simulink model "MenakaModel"  (R2022a)
settings: Solver=ode23tb  StartTime=0.0  StopTime=4  MaxStep=10/(60*24)  RelTol=1e-3
model workspace (MAT data in the model file):
  clima__A_c = 3295.16408265
  clima__A_f = 3100.53942116
  clima__G0 = [0.05; 0.00070738]
  clima__H = 7.9995824611
  clima__T0 = [287.15; 287.15; 287.15; 287.15]
  clima__T_ss = 280.150340169
  clima__alpha_c = 0.0100640347387
  clima__alpha_f = 0.0111385012129
  clima__alpha_i = 0.1
  clima__c_s = [1081 1081]
  clima__cd_c = 8736
  clima__d_c = 1.5
  clima__hour0 = 1
  clima__int_air_speed = 0.5
  clima__l_s = [0.1 0.1]
  clima__lam_s = [2.5 0.85]
  clima__minWindows = 0.299965865643
  clima__rhod_s = [2600 2500]
  clima__tau_c = 1
  crop__A_v = 2080
  crop__C = [0.01 0.001 0.01 0.01]
  crop__C_buf_max = 0.02
  crop__C_wv = 0.2
  crop__Chi_nutrients = [0.015625; 0.0104166666667; 0.00520833333333; 0.00208333333333; 0.00208333333333; 0.00104166666667; 0; 0]
  crop__N = [0; 0; 0; 0; 0; 0; 0; 0]
  crop__R = [0 0 0]
  crop__T_max_v = 40
  crop__T_max_v24 = 27
  crop__T_min_v = 6
  crop__T_min_v24 = 14
  crop__T_sum_end = 1035
  crop__T_v_start_fruit = 1100
  crop__Tsum = 0
  crop__Tv = 288
  crop__b_N_uptake = 0.5
  crop__c_fruit_g = 0.27
  crop__c_fruit_m = 2.3e-07
  crop__c_leaf_g = 0.28
  crop__c_leaf_m = 3.47e-07
  crop__c_stem_g = 0.3
  crop__c_stem_m = 1.47e-07
  crop__fraction_DM = 0.08
  crop__int_air_speed = 0.5
  crop__min_water_capacity = 0.1
  crop__plants_density = 2.1562
  crop__rg_fruit = 2e-07
  crop__rg_leaf = 9.5e-08
  crop__rg_stem = 7.4e-08
  crop__s_buforg_buf = -5000
  crop__s_max_T = 0.5793
  crop__s_max_T24 = 1.3904
  crop__s_min_T = -0.869
  crop__s_min_T24 = -1.1587
  heater__A_e = 0.0001
  heater__A_i = 0.008
  heater__T = 288
  heater__c = 5e-10
  heater__power = 60000000
  screen__Power = 100
  screen__Radthreshold = 900
  screen__beta = 2.23564167038e-14
  screen__gamma_max = 2.26308905438e-14
  screen__velocity = 0.333333333333
  subtrate__C_ws = 0.1
  subtrate__N = [0; 0; 0; 0; 0; 0; 0; 0]
  subtrate__Nmin_subs = 1e-09
  subtrate__Vmax_subs = 10
  subtrate__Vmin_subs = 0.01
  subtrate__sigma_max = 1
  subtrate__sigma_min = 1
  tomato__Cfruit0 = 0.001
  windows__AR = 19.9974923936
  windows__Power = 100
  windows__RadThreshold = 10
  windows__max_night = 10
  windows__tau = 600
undefined symbols (not defined in the file or in its folder): CO2_ppm_ext, Gain_control_Tv_mean, Gain_control_Tv_mean_superior, gain_max_night, GAIN_WIN, Hmax, Hstart, max_night, maxvelocity, RadTh_windows, Radthhold, shift_temp_heat, tau_win, tend_crop1, tend_crop2, tinit_crop1, tinit_crop2, Tmax, Tmax_mean, Tstart, Tven_max, Tven_start, WinAR
libraries: HORTISIM x26, simulink x6
(part 3 of 5)

== system MenakaModel/Control System/Control System Proportional (Ti) + Tmu Windows Relay/Heating Controler/Subsystem2 ==
  " Min" : Inport
  Max : Inport  Port=2
  T : Inport  Port=3
  Divide : Product  Inputs=*/
  Gain : Gain  Gain=0.5
  Gain1 : Gain  Gain=0.5
  Minus : Sum  Inputs=+-
  Minus1 : Sum  Inputs=+-
  Saturation : Saturate  UpperLimit=1  LowerLimit=0
  Sum : Sum  Inputs=|++
  y : Outport
  wires:
  Saturation/1 -> y/1
  Max/1 -> Gain1/1
  T/1 -> Minus/1
  Minus1/1 -> Divide/2
  Minus/1 -> Divide/1
  Divide/1 -> Saturation/1
  " Min"/1 -> Gain/1, Minus1/1
  Gain/1 -> Sum/1
  Gain1/1 -> Sum/2
  Sum/1 -> [Tmu]
  [Tmu] -> Minus1/2, Minus/2

== system MenakaModel/Control System/Control System Proportional (Ti) + Tmu Windows Relay/Screen Controler/Subsystem ==
  In1 : Inport
  Radthhold : Inport  Port=2
  If : If  IfExpression=u1 < 10
  If Action Subsystem : Subsystem  TreatAsAtomicUnit=on
  If Action Subsystem1 : Subsystem  TreatAsAtomicUnit=on
  Merge : Merge
  Smooth Rad : Subsystem
  Out1 : Outport
  wires:
  If/2 -> If Action Subsystem1/Action
  Smooth Rad/1(Out1) -> If/1
  If Action Subsystem1/1(Out1) -> Merge/2
  Merge/1 -> Out1/1
  In1/1 -> If Action Subsystem1/1(EC), Smooth Rad/1(In1)
  If/1 -> If Action Subsystem/Action
  If Action Subsystem/1(Out1) -> Merge/1
  Radthhold/1 -> If Action Subsystem1/2(Radthhold)

== system MenakaModel/Control System/Control System Proportional (Ti) + Tmu Windows Relay/Subsystem/Scalar2Bus  ==
  QV : Inport
  QT : Inport  Port=2
  A : Inport  Port=3
  CC : Inport  Port=4
  Bus Creator : BusCreator  Inputs=4
  CoCl : Outport
  wires:
  A/1 -> Bus Creator/3  "A"
  CC/1 -> Bus Creator/4  "CC"
  QV/1 -> Bus Creator/1  "QV"
  Bus Creator/1 -> CoCl/1
  QT/1 -> Bus Creator/2  "QT"

== system MenakaModel/Control System/Control System Proportional (Ti) + Tmu Windows Relay/Windows Controler/Subsystem ==
  Tstart : Inport
  Ti : Inport  Port=2
  Tmax : Inport  Port=3
  HRInt : Inport  Port=4
  HRStart : Inport  Port=5
  HRMax : Inport  Port=6
  Rad : Inport  Port=7
  Constant : Constant  Value=RadThreshold
  Hum : Saturate  UpperLimit=max_night  LowerLimit=0
  "Selection " : MATLAB Function  TreatAsAtomicUnit=on
  Subsystem : Subsystem
  Temp : Saturate  UpperLimit=100  LowerLimit=0
  Ventilation by Hight Humidity : MATLAB Function  TreatAsAtomicUnit=on
  y : Outport
  wires:
  Ti/1 -> Subsystem/2(Ti)
  Rad/1 -> "Selection "/1(Rad)
  Tstart/1 -> Subsystem/1(Tstart)
  Hum/1 -> "Selection "/3(Humidity)
  HRMax/1 -> Ventilation by Hight Humidity/3(HRMax)
  Tmax/1 -> Subsystem/3(Tmax)
  "Selection "/1(y) -> y/1
  Ventilation by Hight Humidity/1(y) -> Hum/1
  HRStart/1 -> Ventilation by Hight Humidity/2(HRStart)
  Subsystem/1(y) -> Temp/1
  HRInt/1 -> Ventilation by Hight Humidity/1(HRInt)
  Temp/1 -> "Selection "/2(Temperature)
  Constant/1 -> "Selection "/4(Rad_threshold)

== system MenakaModel/Control System/ON//OFF - constant setpoints/Subsystem/Scalar2Bus  ==
  QV : Inport
  QT : Inport  Port=2
  A : Inport  Port=3
  CC : Inport  Port=4
  Bus Creator : BusCreator  Inputs=4
  CoCl : Outport
  wires:
  A/1 -> Bus Creator/3  "A"
  CC/1 -> Bus Creator/4  "CC"
  QV/1 -> Bus Creator/1  "QV"
  Bus Creator/1 -> CoCl/1
  QT/1 -> Bus Creator/2  "QT"

== system MenakaModel/Control System/ON//OFF - constant setpoints/Subsystem1/From Temperature To Heater ST ==
  Tmax : Inport
  Tmin : Inport  Port=2
  Tmean : Inport  Port=3
  Constant1 : Constant  Value=shift_temp_heat
  Constant2 : Constant  Value=shift_temp_heat
  Integrator : Integrator  InitialConditionSource=external
  Minus2 : Sum  Inputs=+-
  Sum : Sum  Inputs=|++
  Sum1 : Sum  Inputs=|++
  Tmax_h : Outport
  Tstart_h : Outport  Port=2
  Tplus : Outport  Port=3
  Tminus : Outport  Port=4
  T_mu_mu : Outport  Port=5
  tag scope: Tmax_heater=global, Tmin_heater=global
  wires:
  Tmax/1 -> Sum/1
  Sum/1 -> [Tmax_heater], Tmax_h/1
  Tmin/1 -> Sum1/1
  Sum1/1 -> Tstart_h/1, [Tmin_heater]
  Constant1/1 -> Sum/2
  Constant2/1 -> Sum1/2
  Integrator/1 -> Minus2/2, T_mu_mu/1
  Minus2/1 -> Integrator/1
  Tmean/1 -> Integrator/2, Minus2/1

== system MenakaModel/Control System/ON//OFF - constant setpoints/Subsystem1/Heating Controler ==
  In Bus Element : Inport  PortName=EC  Element=Temp
  In Bus Element1 : Inport  Port=2  PortName=IC  Element=Temp.Tair
  u : Inport  Port=3
  Gain : Gain  Gain=power
  Integrator : Integrator  InitialCondition=T  AbsoluteTolerance=0.001
  Sec2Days : Gain  Gain=24*3600
  Subsystem : Subsystem
  Heater : Outport  Unit=J
  Consumptions : Outport  Port=2
  State : Outport  Port=3
  wires:
  Gain/1 -> Consumptions/1, Subsystem/2(Q_h)  "Q_h"
  u/1 -> Gain/1  "Control"
  Sec2Days/1 -> Integrator/1
  In Bus Element1/1 -> Subsystem/1(T_i)
  In Bus Element/1 -> Subsystem/3(T_e)
  Subsystem/1(QV_h_i) -> Heater/1  "QV_h_i"
  Subsystem/2(dT_h_dt) -> Sec2Days/1
  Integrator/1 -> State/1, Subsystem/4(Th)  "Th"

== system MenakaModel/Control System/ON//OFF - constant setpoints/Subsystem1/Subsystem2 ==
  Max : Inport
  " Min" : Inport  Port=2
  T : Inport  Port=3
  If : If  NumInputs=3  IfExpression=u2 > u1  ElseIfExpressions=u2 < u3
  If Action Subsystem : Subsystem  TreatAsAtomicUnit=on
  If Action Subsystem1 : Subsystem  TreatAsAtomicUnit=on
  If Action Subsystem2 : Subsystem  TreatAsAtomicUnit=on
  Memory : Memory  InheritSampleTime=on
  Merge : Merge  Inputs=3
  y : Outport
  wires:
  " Min"/1 -> If/3
  If Action Subsystem/1(Out1) -> Merge/1
  Max/1 -> If/1
  If/1 -> If Action Subsystem/Action
  Merge/1 -> y/1, Memory/1
  Memory/1 -> If Action Subsystem2/1(In1)
  If/2 -> If Action Subsystem1/Action
  T/1 -> If/2
  If Action Subsystem1/1(Out1) -> Merge/2
  If/3 -> If Action Subsystem2/Action
  If Action Subsystem2/1(Out1) -> Merge/3

== system MenakaModel/Control System/ON//OFF - constant setpoints/Subsystem1/Windows Controler ==
  note: Subsystem1
  In Bus Element : Inport  PortName=IC  Element=QS.R_int
  In Bus Element1 : Inport  PortName=IC  Element=Temp.Tair
  In Bus Element2 : Inport  PortName=IC  Element=Gas.HRInt
  Tstart : Inport  Port=2
  Tmax : Inport  Port=3
  Hstart : Inport  Port=4
  Hmax : Inport  Port=5
  max_night : Inport  Port=6
  Abs : Abs  ZeroCross=off  SaturateOnIntegerOverflow=off
  Bus Creator : BusCreator  Inputs=2
  Constant : Constant  Value=AR
  Gain : Gain  Gain=100/tau
  Gain1 : Gain  Gain=Power
  Integrator : Integrator
  Minus : Sum  Inputs=+-
  Sec2Days : Gain  Gain=24*3600
  Subsystem : Subsystem
      settings: PortSchema="{\"entries\":[{\"content\":{\"sides\":[{\"content\":{\"connectorIds\":[\"In1\",\"In2\",\"In3\",\"In4\",\"In5\",\"In6\"]},\"type\":\"ConnectorPlacement.EquallySpacedRectSide\",\"uuid\":\"18d05740-181f-409c-94ea-b42b6e57ea74\"},{\"content\":{\"connectorIds\":[\"Out1\"],\"side\":\"RIGHT\"},\"type\":\"ConnectorPlacement.EquallySpacedRectSide\",\"uuid\":\"978406c3-d241-44cd-a3e7-fe734e3a171e\"},{\"content\":{\"connectorIds\":[\"In7\",\"In8\"],\"side\":\"TOP\"},\"type\":\"ConnectorPlacement.EquallySpacedRectSide\",\"uuid\":\"b3c10a0e-c6d9-4444-97f2-9f0c7dea8ec9\"}]},\"type\":\"ConnectorPlacement.EquallySpacedConnector\",\"uuid\":\"429bf3f5-5806-495e-b66b-96810540e6d1\"}],\"packageUris\":[\"http://schema.mathworks.com/mf0/Connector/R2020b\"],\"version\":\"1.0\"}"
  Tanh : Trigonometry  Operator=tanh
  Windows : Outport
  Consumptions : Outport  Port=2
  wires:
  Tstart/1 -> Subsystem/1(Tstart)
  In Bus Element1/1 -> Subsystem/2(Ti)
  Tmax/1 -> Subsystem/3(Tmax)
  Integrator/1 -> Bus Creator/1, Minus/2  "value"
  In Bus Element2/1 -> Subsystem/4(HRInt)
  Hstart/1 -> Subsystem/5(HRStart)
  In Bus Element/1 -> Subsystem/7(Rad)
  Hmax/1 -> Subsystem/6(HRMax)
  Subsystem/1(y) -> Minus/1
  Sec2Days/1 -> Integrator/1
  Gain1/1 -> Consumptions/1  "Power"
  Abs/1 -> Gain1/1
  Gain/1 -> Abs/1, Sec2Days/1
  Tanh/1 -> Gain/1
  Minus/1 -> Tanh/1
  Bus Creator/1 -> Windows/1
  Constant/1 -> Bus Creator/2  "AR"
  max_night/1 -> Subsystem/8(max_night)

== system MenakaModel/Control System/PID - const st - Ti mesure - Dynamics ST/Subsystem/Scalar2Bus  ==
  QV : Inport
  QT : Inport  Port=2
  A : Inport  Port=3
  CC : Inport  Port=4
  Bus Creator : BusCreator  Inputs=4
  CoCl : Outport
  wires:
  A/1 -> Bus Creator/3  "A"
  CC/1 -> Bus Creator/4  "CC"
  QV/1 -> Bus Creator/1  "QV"
  Bus Creator/1 -> CoCl/1
  QT/1 -> Bus Creator/2  "QT"

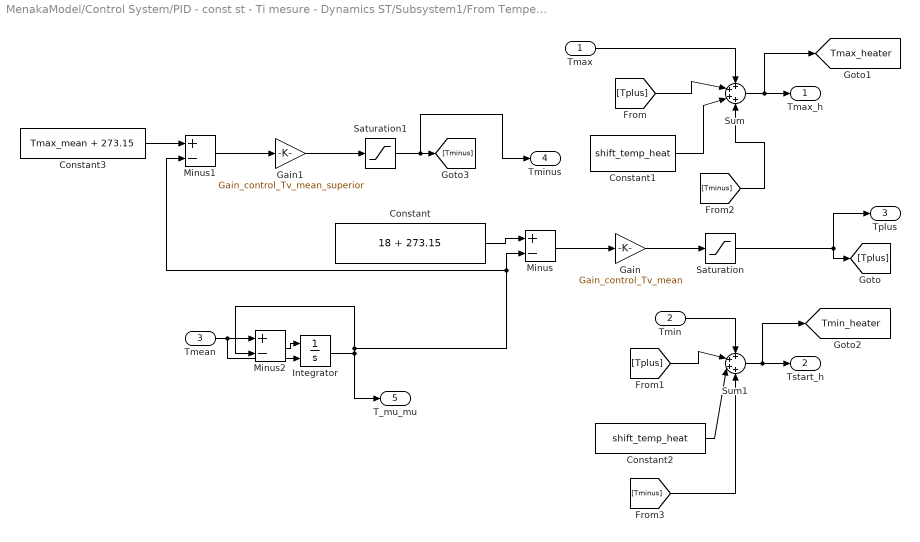
== system MenakaModel/Control System/PID - const st - Ti mesure - Dynamics ST/Subsystem1/From Temperature To Heater ST ==
  Tmax : Inport
  Tmin : Inport  Port=2
  Tmean : Inport  Port=3
  Constant : Constant  Value=18 + 273.15
  Constant1 : Constant  Value=shift_temp_heat
  Constant2 : Constant  Value=shift_temp_heat
  Constant3 : Constant  Value=Tmax_mean + 273.15
  Gain : Gain  Gain=Gain_control_Tv_mean
  Gain1 : Gain  Gain=Gain_control_Tv_mean_superior
  Integrator : Integrator  InitialConditionSource=external
  Minus : Sum  Inputs=+-
  Minus1 : Sum  Inputs=+-
  Minus2 : Sum  Inputs=+-
  Saturation : Saturate  UpperLimit=inf  LowerLimit=0
  Saturation1 : Saturate  UpperLimit=0  LowerLimit=-inf
  Sum : Sum  Inputs=++++
  Sum1 : Sum  Inputs=++++
  Tmax_h : Outport
  Tstart_h : Outport  Port=2
  Tplus : Outport  Port=3
  Tminus : Outport  Port=4
  T_mu_mu : Outport  Port=5
  tag scope: Tmax_heater=global, Tmin_heater=global
  wires:
  Tmin/1 -> Sum1/1
  Tmean/1 -> Integrator/2, Minus2/1
  Gain1/1 -> Saturation1/1
  Saturation/1 -> [Tplus], Tplus/1
  Saturation1/1 -> Tminus/1, [Tminus]
  Constant3/1 -> Minus1/1
  [Tplus] -> Sum/2
  [Tplus] -> Sum1/2
  Minus/1 -> Gain/1
  Constant2/1 -> Sum1/3
  Constant1/1 -> Sum/3
  Sum/1 -> [Tmax_heater], Tmax_h/1
  Gain/1 -> Saturation/1
  Constant/1 -> Minus/1
  Integrator/1 -> Minus1/2, Minus/2, Minus2/2, T_mu_mu/1
  Minus1/1 -> Gain1/1
  Sum1/1 -> [Tmin_heater], Tstart_h/1
  Tmax/1 -> Sum/1
  [Tminus] -> Sum/4
  [Tminus] -> Sum1/4
  Minus2/1 -> Integrator/1

== system MenakaModel/Control System/PID - const st - Ti mesure - Dynamics ST/Subsystem1/Heating Controler ==
  In Bus Element : Inport  PortName=EC  Element=Temp
  In Bus Element1 : Inport  Port=2  PortName=IC  Element=Temp.Tair
  u : Inport  Port=3
  Gain : Gain  Gain=power
  Integrator : Integrator  InitialCondition=T  AbsoluteTolerance=0.001
  Sec2Days : Gain  Gain=24*3600
  Subsystem : Subsystem
  Heater : Outport  Unit=J
  Consumptions : Outport  Port=2
  State : Outport  Port=3
  wires:
  Gain/1 -> Consumptions/1, Subsystem/2(Q_h)  "Q_h"
  u/1 -> Gain/1  "Control"
  Sec2Days/1 -> Integrator/1
  In Bus Element1/1 -> Subsystem/1(T_i)
  In Bus Element/1 -> Subsystem/3(T_e)
  Subsystem/1(QV_h_i) -> Heater/1  "QV_h_i"
  Subsystem/2(dT_h_dt) -> Sec2Days/1
  Integrator/1 -> State/1, Subsystem/4(Th)  "Th"

== system MenakaModel/Control System/PID - const st - Ti mesure - Dynamics ST/Subsystem1/Subsystem2 ==
  Max : Inport
  " Min" : Inport  Port=2
  T : Inport  Port=3
  IC : Inport  Port=4
  PI : Subsystem  VariantControl=Choice_1
  Subsystem2 : Subsystem  VariantControl=Choice
      settings: PortSchema="{\"entries\":[{\"content\":{\"sides\":[{\"content\":{\"connectorIds\":[\"In1\",\"In2\"]},\"type\":\"ConnectorPlacement.EquallySpacedRectSide\",\"uuid\":\"76a0539e-cd8b-47df-82d9-61971d3be914\"},{\"content\":{\"connectorIds\":[\"Out1\"],\"side\":\"RIGHT\"},\"type\":\"ConnectorPlacement.EquallySpacedRectSide\",\"uuid\":\"93f2ebb7-6ab4-4fcc-bc7a-3583f1db6e8e\"},{\"content\":{\"connectorIds\":[],\"side\":\"TOP\"},\"type\":\"ConnectorPlacement.EquallySpacedRectSide\",\"uuid\":\"b50a0ff6-3876-4dcb-8bb9-79340929aa80\"},{\"content\":{\"connectorIds\":[\"In3\",\"In4\"],\"side\":\"BOTTOM\"},\"type\":\"ConnectorPlacement.EquallySpacedRectSide\",\"uuid\":\"63f2a7a5-83ef-48e2-af90-7d61b47411e6\"}]},\"type\":\"ConnectorPlacement.EquallySpacedConnector\",\"uuid\":\"d97900b9-3143-4b55-b66d-f73dd0302926\"}],\"packageUris\":[\"http://schema.mathworks.com/mf0/Connector/R2020b\"],\"version\":\"1.0\"}"
  y : Outport

== system MenakaModel/Control System/PID - const st - Ti mesure - Dynamics ST/Subsystem1/Sunset Sunrise ==
  Rad : Inport
  Constant4 : Constant  Value=100
  Gain : Gain  Gain=10
  Minus : Sum  Inputs=+-
  Tan : Trigonometry  Operator=tanh
  Out1 : Outport
  wires:
  Constant4/1 -> Minus/2
  Tan/1 -> Out1/1
  Gain/1 -> Tan/1
  Minus/1 -> Gain/1
  Rad/1 -> Minus/1

== system MenakaModel/Control System/PID - const st - Ti mesure - Dynamics ST/Subsystem1/Triggered Subsystem ==
  Rad : Inport
  <Tsum> : Inport  Port=2
  Trigger : TriggerPort  TriggerType=either  VariantControl=(inherit)  InitialTriggerSignalState=positive
  Constant : Constant  Value=100
  MATLAB Function : MATLAB Function  TreatAsAtomicUnit=on
  T_min : Outport
  T_opt_min : Outport  Port=2
  T_opt_max : Outport  Port=3
  Tmax : Outport  Port=4
  wires:
  <Tsum>/1 -> MATLAB Function/1(Tsum)
  Rad/1 -> MATLAB Function/2(Rad)
  Constant/1 -> MATLAB Function/3(THRad)
  MATLAB Function/1(T_min) -> T_min/1
  MATLAB Function/2(T_opt_min) -> T_opt_min/1
  MATLAB Function/3(T_opt_max) -> T_opt_max/1
  MATLAB Function/4(Tmax) -> Tmax/1

== system MenakaModel/Control System/PID - const st - Ti mesure - Dynamics ST/Subsystem1/Windows Controler ==
  note: Subsystem1
  In Bus Element : Inport  PortName=IC  Element=QS.R_int
  In Bus Element1 : Inport  PortName=IC  Element=Temp.Tair
  In Bus Element2 : Inport  PortName=IC  Element=Gas.HRInt
  Tstart : Inport  Port=2
  Tmax : Inport  Port=3
  Hstart : Inport  Port=4
  Hmax : Inport  Port=5
  max_night : Inport  Port=6
  Abs : Abs  ZeroCross=off  SaturateOnIntegerOverflow=off
  Bus Creator : BusCreator  Inputs=2
  Constant : Constant  Value=AR
  Gain : Gain  Gain=100/tau
  Gain1 : Gain  Gain=Power
  Integrator : Integrator
  Minus : Sum  Inputs=+-
  Sec2Days : Gain  Gain=24*3600
  Subsystem : Subsystem
      settings: PortSchema="{\"entries\":[{\"content\":{\"sides\":[{\"content\":{\"connectorIds\":[\"In1\",\"In2\",\"In3\",\"In4\",\"In5\",\"In6\"]},\"type\":\"ConnectorPlacement.EquallySpacedRectSide\",\"uuid\":\"18d05740-181f-409c-94ea-b42b6e57ea74\"},{\"content\":{\"connectorIds\":[\"Out1\"],\"side\":\"RIGHT\"},\"type\":\"ConnectorPlacement.EquallySpacedRectSide\",\"uuid\":\"978406c3-d241-44cd-a3e7-fe734e3a171e\"},{\"content\":{\"connectorIds\":[\"In7\",\"In8\"],\"side\":\"TOP\"},\"type\":\"ConnectorPlacement.EquallySpacedRectSide\",\"uuid\":\"b3c10a0e-c6d9-4444-97f2-9f0c7dea8ec9\"}]},\"type\":\"ConnectorPlacement.EquallySpacedConnector\",\"uuid\":\"429bf3f5-5806-495e-b66b-96810540e6d1\"}],\"packageUris\":[\"http://schema.mathworks.com/mf0/Connector/R2020b\"],\"version\":\"1.0\"}"
  Tanh : Trigonometry  Operator=tanh
  Windows : Outport
  Consumptions : Outport  Port=2
  wires:
  Tstart/1 -> Subsystem/1(Tstart)
  In Bus Element1/1 -> Subsystem/2(Ti)
  Tmax/1 -> Subsystem/3(Tmax)
  Integrator/1 -> Bus Creator/1, Minus/2  "value"
  In Bus Element2/1 -> Subsystem/4(HRInt)
  Hstart/1 -> Subsystem/5(HRStart)
  In Bus Element/1 -> Subsystem/7(Rad)
  Hmax/1 -> Subsystem/6(HRMax)
  Subsystem/1(y) -> Minus/1
  Sec2Days/1 -> Integrator/1
  Gain1/1 -> Consumptions/1  "Power"
  Abs/1 -> Gain1/1
  Gain/1 -> Abs/1, Sec2Days/1
  Tanh/1 -> Gain/1
  Minus/1 -> Tanh/1
  Bus Creator/1 -> Windows/1
  Constant/1 -> Bus Creator/2  "AR"
  max_night/1 -> Subsystem/8(max_night)

== system MenakaModel/Control System/PID - constant setpoints/Subsystem/Scalar2Bus  ==
  QV : Inport
  QT : Inport  Port=2
  A : Inport  Port=3
  CC : Inport  Port=4
  Bus Creator : BusCreator  Inputs=4
  CoCl : Outport
  wires:
  A/1 -> Bus Creator/3  "A"
  CC/1 -> Bus Creator/4  "CC"
  QV/1 -> Bus Creator/1  "QV"
  Bus Creator/1 -> CoCl/1
  QT/1 -> Bus Creator/2  "QT"

== system MenakaModel/Control System/PID - constant setpoints/Subsystem1/From Temperature To Heater ST ==
  Tmax : Inport
  Tmin : Inport  Port=2
  Tmean : Inport  Port=3
  Constant1 : Constant  Value=shift_temp_heat
  Constant2 : Constant  Value=shift_temp_heat
  Integrator : Integrator  InitialConditionSource=external
  Minus2 : Sum  Inputs=+-
  Sum : Sum  Inputs=|++
  Sum1 : Sum  Inputs=|++
  Tmax_h : Outport
  Tstart_h : Outport  Port=2
  Tplus : Outport  Port=3
  Tminus : Outport  Port=4
  T_mu_mu : Outport  Port=5
  tag scope: Tmax_heater=global, Tmin_heater=global
  wires:
  Tmax/1 -> Sum/1
  Sum/1 -> [Tmax_heater], Tmax_h/1
  Tmin/1 -> Sum1/1
  Sum1/1 -> Tstart_h/1, [Tmin_heater]
  Constant1/1 -> Sum/2
  Constant2/1 -> Sum1/2
  Integrator/1 -> Minus2/2, T_mu_mu/1
  Minus2/1 -> Integrator/1
  Tmean/1 -> Integrator/2, Minus2/1

== system MenakaModel/Control System/PID - constant setpoints/Subsystem1/Heating Controler ==
  In Bus Element : Inport  PortName=EC  Element=Temp
  In Bus Element1 : Inport  Port=2  PortName=IC  Element=Temp.Tair
  u : Inport  Port=3
  Gain : Gain  Gain=power
  Integrator : Integrator  InitialCondition=T  AbsoluteTolerance=0.001
  Sec2Days : Gain  Gain=24*3600
  Subsystem : Subsystem
  Heater : Outport  Unit=J
  Consumptions : Outport  Port=2
  State : Outport  Port=3
  wires:
  Gain/1 -> Consumptions/1, Subsystem/2(Q_h)  "Q_h"
  u/1 -> Gain/1  "Control"
  Sec2Days/1 -> Integrator/1
  In Bus Element1/1 -> Subsystem/1(T_i)
  In Bus Element/1 -> Subsystem/3(T_e)
  Subsystem/1(QV_h_i) -> Heater/1  "QV_h_i"
  Subsystem/2(dT_h_dt) -> Sec2Days/1
  Integrator/1 -> State/1, Subsystem/4(Th)  "Th"

== system MenakaModel/Control System/PID - constant setpoints/Subsystem1/Subsystem2 ==
  Max : Inport
  " Min" : Inport  Port=2
  T : Inport  Port=3
  In Bus Element : Inport  Port=4  PortName=IC  Element=Temp.Tair
  Gain : Gain
  Gain1 : Gain  Gain=0.5
  Minus : Sum  Inputs=+-
  Saturation : Saturate  UpperLimit=1  LowerLimit=0
  Sum : Sum  Inputs=|++
  y : Outport
  wires:
  Max/1 -> Gain1/1
  Gain/1 -> Saturation/1
  Minus/1 -> Gain/1
  Saturation/1 -> y/1
  Gain1/1 -> Sum/1
  T/1 -> Minus/2
  " Min"/1 -> Minus/1

== system MenakaModel/Control System/PID - constant setpoints/Subsystem1/Sunset Sunrise ==
  Rad : Inport
  Constant4 : Constant  Value=100
  Gain : Gain  Gain=10
  Minus : Sum  Inputs=+-
  Tan : Trigonometry  Operator=tanh
  Out1 : Outport
  wires:
  Constant4/1 -> Minus/2
  Tan/1 -> Out1/1
  Gain/1 -> Tan/1
  Minus/1 -> Gain/1
  Rad/1 -> Minus/1

== system MenakaModel/Control System/PID - constant setpoints/Subsystem1/Triggered Subsystem ==
  Rad : Inport
  <Tsum> : Inport  Port=2
  Trigger : TriggerPort  TriggerType=either  VariantControl=(inherit)  InitialTriggerSignalState=positive
  Constant : Constant  Value=100
  MATLAB Function : MATLAB Function  TreatAsAtomicUnit=on
  T_min : Outport
  T_opt_min : Outport  Port=2
  T_opt_max : Outport  Port=3
  Tmax : Outport  Port=4
  wires:
  <Tsum>/1 -> MATLAB Function/1(Tsum)
  Rad/1 -> MATLAB Function/2(Rad)
  Constant/1 -> MATLAB Function/3(THRad)
  MATLAB Function/1(T_min) -> T_min/1
  MATLAB Function/2(T_opt_min) -> T_opt_min/1
  MATLAB Function/3(T_opt_max) -> T_opt_max/1
  MATLAB Function/4(Tmax) -> Tmax/1

== system MenakaModel/Control System/PID - constant setpoints/Subsystem1/Windows Controler ==
  note: Subsystem1
  In Bus Element : Inport  PortName=IC  Element=QS.R_int
  In Bus Element1 : Inport  PortName=IC  Element=Temp.Tair
  In Bus Element2 : Inport  PortName=IC  Element=Gas.HRInt
  Tstart : Inport  Port=2
  Tmax : Inport  Port=3
  Hstart : Inport  Port=4
  Hmax : Inport  Port=5
  max_night : Inport  Port=6
  Abs : Abs  ZeroCross=off  SaturateOnIntegerOverflow=off
  Bus Creator : BusCreator  Inputs=2
  Constant : Constant  Value=AR
  Gain : Gain  Gain=100/tau
  Gain1 : Gain  Gain=Power
  Integrator : Integrator
  Minus : Sum  Inputs=+-
  Sec2Days : Gain  Gain=24*3600
  Subsystem : Subsystem
      settings: PortSchema="{\"entries\":[{\"content\":{\"sides\":[{\"content\":{\"connectorIds\":[\"In1\",\"In2\",\"In3\",\"In4\",\"In5\",\"In6\"]},\"type\":\"ConnectorPlacement.EquallySpacedRectSide\",\"uuid\":\"18d05740-181f-409c-94ea-b42b6e57ea74\"},{\"content\":{\"connectorIds\":[\"Out1\"],\"side\":\"RIGHT\"},\"type\":\"ConnectorPlacement.EquallySpacedRectSide\",\"uuid\":\"978406c3-d241-44cd-a3e7-fe734e3a171e\"},{\"content\":{\"connectorIds\":[\"In7\",\"In8\"],\"side\":\"TOP\"},\"type\":\"ConnectorPlacement.EquallySpacedRectSide\",\"uuid\":\"b3c10a0e-c6d9-4444-97f2-9f0c7dea8ec9\"}]},\"type\":\"ConnectorPlacement.EquallySpacedConnector\",\"uuid\":\"429bf3f5-5806-495e-b66b-96810540e6d1\"}],\"packageUris\":[\"http://schema.mathworks.com/mf0/Connector/R2020b\"],\"version\":\"1.0\"}"
  Tanh : Trigonometry  Operator=tanh
  Windows : Outport
  Consumptions : Outport  Port=2
  wires:
  Tstart/1 -> Subsystem/1(Tstart)
  In Bus Element1/1 -> Subsystem/2(Ti)
  Tmax/1 -> Subsystem/3(Tmax)
  Integrator/1 -> Bus Creator/1, Minus/2  "value"
  In Bus Element2/1 -> Subsystem/4(HRInt)
  Hstart/1 -> Subsystem/5(HRStart)
  In Bus Element/1 -> Subsystem/7(Rad)
  Hmax/1 -> Subsystem/6(HRMax)
  Subsystem/1(y) -> Minus/1
  Sec2Days/1 -> Integrator/1
  Gain1/1 -> Consumptions/1  "Power"
  Abs/1 -> Gain1/1
  Gain/1 -> Abs/1, Sec2Days/1
  Tanh/1 -> Gain/1
  Minus/1 -> Tanh/1
  Bus Creator/1 -> Windows/1
  Constant/1 -> Bus Creator/2  "AR"
  max_night/1 -> Subsystem/8(max_night)

== system MenakaModel/Control System/PID - constant setpoints - Ti measure/Subsystem/Scalar2Bus  ==
  QV : Inport
  QT : Inport  Port=2
  A : Inport  Port=3
  CC : Inport  Port=4
  Bus Creator : BusCreator  Inputs=4
  CoCl : Outport
  wires:
  A/1 -> Bus Creator/3  "A"
  CC/1 -> Bus Creator/4  "CC"
  QV/1 -> Bus Creator/1  "QV"
  Bus Creator/1 -> CoCl/1
  QT/1 -> Bus Creator/2  "QT"

== system MenakaModel/Control System/PID - constant setpoints - Ti measure/Subsystem1/From Temperature To Heater ST ==
  Tmax : Inport
  Tmin : Inport  Port=2
  Tmean : Inport  Port=3
  Constant1 : Constant  Value=shift_temp_heat
  Constant2 : Constant  Value=shift_temp_heat
  Integrator : Integrator  InitialConditionSource=external
  Minus2 : Sum  Inputs=+-
  Sum : Sum  Inputs=|++
  Sum1 : Sum  Inputs=|++
  Tmax_h : Outport
  Tstart_h : Outport  Port=2
  Tplus : Outport  Port=3
  Tminus : Outport  Port=4
  T_mu_mu : Outport  Port=5
  tag scope: Tmax_heater=global, Tmin_heater=global
  wires:
  Tmax/1 -> Sum/1
  Sum/1 -> [Tmax_heater], Tmax_h/1
  Tmin/1 -> Sum1/1
  Sum1/1 -> Tstart_h/1, [Tmin_heater]
  Constant1/1 -> Sum/2
  Constant2/1 -> Sum1/2
  Integrator/1 -> Minus2/2, T_mu_mu/1
  Minus2/1 -> Integrator/1
  Tmean/1 -> Integrator/2, Minus2/1

== system MenakaModel/Control System/PID - constant setpoints - Ti measure/Subsystem1/Heating Controler ==
  In Bus Element : Inport  PortName=EC  Element=Temp
  In Bus Element1 : Inport  Port=2  PortName=IC  Element=Temp.Tair
  u : Inport  Port=3
  Gain : Gain  Gain=power
  Integrator : Integrator  InitialCondition=T  AbsoluteTolerance=0.001
  Sec2Days : Gain  Gain=24*3600
  Subsystem : Subsystem
  Heater : Outport  Unit=J
  Consumptions : Outport  Port=2
  State : Outport  Port=3
  wires:
  Gain/1 -> Consumptions/1, Subsystem/2(Q_h)  "Q_h"
  u/1 -> Gain/1  "Control"
  Sec2Days/1 -> Integrator/1
  In Bus Element1/1 -> Subsystem/1(T_i)
  In Bus Element/1 -> Subsystem/3(T_e)
  Subsystem/1(QV_h_i) -> Heater/1  "QV_h_i"
  Subsystem/2(dT_h_dt) -> Sec2Days/1
  Integrator/1 -> State/1, Subsystem/4(Th)  "Th"

== system MenakaModel/Control System/PID - constant setpoints - Ti measure/Subsystem1/Subsystem2 ==
  Max : Inport
  " Min" : Inport  Port=2
  T : Inport  Port=3
  IC : Inport  Port=4
  PI : Subsystem  VariantControl=Choice_1
  Subsystem2 : Subsystem  VariantControl=Choice
      settings: PortSchema="{\"entries\":[{\"content\":{\"sides\":[{\"content\":{\"connectorIds\":[\"In1\",\"In2\"]},\"type\":\"ConnectorPlacement.EquallySpacedRectSide\",\"uuid\":\"76a0539e-cd8b-47df-82d9-61971d3be914\"},{\"content\":{\"connectorIds\":[\"Out1\"],\"side\":\"RIGHT\"},\"type\":\"ConnectorPlacement.EquallySpacedRectSide\",\"uuid\":\"93f2ebb7-6ab4-4fcc-bc7a-3583f1db6e8e\"},{\"content\":{\"connectorIds\":[],\"side\":\"TOP\"},\"type\":\"ConnectorPlacement.EquallySpacedRectSide\",\"uuid\":\"b50a0ff6-3876-4dcb-8bb9-79340929aa80\"},{\"content\":{\"connectorIds\":[\"In3\",\"In4\"],\"side\":\"BOTTOM\"},\"type\":\"ConnectorPlacement.EquallySpacedRectSide\",\"uuid\":\"63f2a7a5-83ef-48e2-af90-7d61b47411e6\"}]},\"type\":\"ConnectorPlacement.EquallySpacedConnector\",\"uuid\":\"d97900b9-3143-4b55-b66d-f73dd0302926\"}],\"packageUris\":[\"http://schema.mathworks.com/mf0/Connector/R2020b\"],\"version\":\"1.0\"}"
  y : Outport

== system MenakaModel/Control System/PID - constant setpoints - Ti measure/Subsystem1/Sunset Sunrise ==
  Rad : Inport
  Constant4 : Constant  Value=100
  Gain : Gain  Gain=10
  Minus : Sum  Inputs=+-
  Tan : Trigonometry  Operator=tanh
  Out1 : Outport
  wires:
  Constant4/1 -> Minus/2
  Tan/1 -> Out1/1
  Gain/1 -> Tan/1
  Minus/1 -> Gain/1
  Rad/1 -> Minus/1

== system MenakaModel/Control System/PID - constant setpoints - Ti measure/Subsystem1/Triggered Subsystem ==
  Rad : Inport
  <Tsum> : Inport  Port=2
  Trigger : TriggerPort  TriggerType=either  VariantControl=(inherit)  InitialTriggerSignalState=positive
  Constant : Constant  Value=100
  MATLAB Function : MATLAB Function  TreatAsAtomicUnit=on
  T_min : Outport
  T_opt_min : Outport  Port=2
  T_opt_max : Outport  Port=3
  Tmax : Outport  Port=4
  wires:
  <Tsum>/1 -> MATLAB Function/1(Tsum)
  Rad/1 -> MATLAB Function/2(Rad)
  Constant/1 -> MATLAB Function/3(THRad)
  MATLAB Function/1(T_min) -> T_min/1
  MATLAB Function/2(T_opt_min) -> T_opt_min/1
  MATLAB Function/3(T_opt_max) -> T_opt_max/1
  MATLAB Function/4(Tmax) -> Tmax/1

== system MenakaModel/Control System/PID - constant setpoints - Ti measure/Subsystem1/Windows Controler ==
  note: Subsystem1
  In Bus Element : Inport  PortName=IC  Element=QS.R_int
  In Bus Element1 : Inport  PortName=IC  Element=Temp.Tair
  In Bus Element2 : Inport  PortName=IC  Element=Gas.HRInt
  Tstart : Inport  Port=2
  Tmax : Inport  Port=3
  Hstart : Inport  Port=4
  Hmax : Inport  Port=5
  max_night : Inport  Port=6
  Abs : Abs  ZeroCross=off  SaturateOnIntegerOverflow=off
  Bus Creator : BusCreator  Inputs=2
  Constant : Constant  Value=AR
  Gain : Gain  Gain=100/tau
  Gain1 : Gain  Gain=Power
  Integrator : Integrator
  Minus : Sum  Inputs=+-
  Sec2Days : Gain  Gain=24*3600
  Subsystem : Subsystem
      settings: PortSchema="{\"entries\":[{\"content\":{\"sides\":[{\"content\":{\"connectorIds\":[\"In1\",\"In2\",\"In3\",\"In4\",\"In5\",\"In6\"]},\"type\":\"ConnectorPlacement.EquallySpacedRectSide\",\"uuid\":\"18d05740-181f-409c-94ea-b42b6e57ea74\"},{\"content\":{\"connectorIds\":[\"Out1\"],\"side\":\"RIGHT\"},\"type\":\"ConnectorPlacement.EquallySpacedRectSide\",\"uuid\":\"978406c3-d241-44cd-a3e7-fe734e3a171e\"},{\"content\":{\"connectorIds\":[\"In7\",\"In8\"],\"side\":\"TOP\"},\"type\":\"ConnectorPlacement.EquallySpacedRectSide\",\"uuid\":\"b3c10a0e-c6d9-4444-97f2-9f0c7dea8ec9\"}]},\"type\":\"ConnectorPlacement.EquallySpacedConnector\",\"uuid\":\"429bf3f5-5806-495e-b66b-96810540e6d1\"}],\"packageUris\":[\"http://schema.mathworks.com/mf0/Connector/R2020b\"],\"version\":\"1.0\"}"
  Tanh : Trigonometry  Operator=tanh
  Windows : Outport
  Consumptions : Outport  Port=2
  wires:
  Tstart/1 -> Subsystem/1(Tstart)
  In Bus Element1/1 -> Subsystem/2(Ti)
  Tmax/1 -> Subsystem/3(Tmax)
  Integrator/1 -> Bus Creator/1, Minus/2  "value"
  In Bus Element2/1 -> Subsystem/4(HRInt)
  Hstart/1 -> Subsystem/5(HRStart)
  In Bus Element/1 -> Subsystem/7(Rad)
  Hmax/1 -> Subsystem/6(HRMax)
  Subsystem/1(y) -> Minus/1
  Sec2Days/1 -> Integrator/1
  Gain1/1 -> Consumptions/1  "Power"
  Abs/1 -> Gain1/1
  Gain/1 -> Abs/1, Sec2Days/1
  Tanh/1 -> Gain/1
  Minus/1 -> Tanh/1
  Bus Creator/1 -> Windows/1
  Constant/1 -> Bus Creator/2  "AR"
  max_night/1 -> Subsystem/8(max_night)

== system MenakaModel/Control System/PID-set-points/Subsystem/Scalar2Bus  ==
  QV : Inport
  QT : Inport  Port=2
  A : Inport  Port=3
  CC : Inport  Port=4
  Bus Creator : BusCreator  Inputs=4
  CoCl : Outport
  wires:
  A/1 -> Bus Creator/3  "A"
  CC/1 -> Bus Creator/4  "CC"
  QV/1 -> Bus Creator/1  "QV"
  Bus Creator/1 -> CoCl/1
  QT/1 -> Bus Creator/2  "QT"

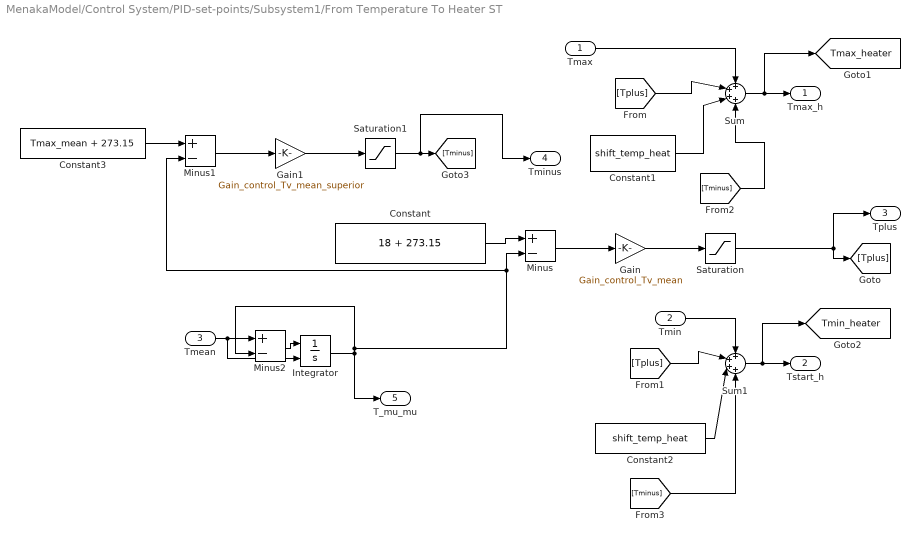
== system MenakaModel/Control System/PID-set-points/Subsystem1/From Temperature To Heater ST ==
  Tmax : Inport
  Tmin : Inport  Port=2
  Tmean : Inport  Port=3
  Constant : Constant  Value=18 + 273.15
  Constant1 : Constant  Value=shift_temp_heat
  Constant2 : Constant  Value=shift_temp_heat
  Constant3 : Constant  Value=Tmax_mean + 273.15
  Gain : Gain  Gain=Gain_control_Tv_mean
  Gain1 : Gain  Gain=Gain_control_Tv_mean_superior
  Integrator : Integrator  InitialConditionSource=external
  Minus : Sum  Inputs=+-
  Minus1 : Sum  Inputs=+-
  Minus2 : Sum  Inputs=+-
  Saturation : Saturate  UpperLimit=inf  LowerLimit=0
  Saturation1 : Saturate  UpperLimit=0  LowerLimit=-inf
  Sum : Sum  Inputs=++++
  Sum1 : Sum  Inputs=++++
  Tmax_h : Outport
  Tstart_h : Outport  Port=2
  Tplus : Outport  Port=3
  Tminus : Outport  Port=4
  T_mu_mu : Outport  Port=5
  tag scope: Tmax_heater=global, Tmin_heater=global
  wires:
  Constant/1 -> Minus/1
  Minus/1 -> Gain/1
  Tmax/1 -> Sum/1
  Sum/1 -> [Tmax_heater], Tmax_h/1
  Saturation/1 -> [Tplus], Tplus/1
  Tmin/1 -> Sum1/1
  Sum1/1 -> [Tmin_heater], Tstart_h/1
  [Tplus] -> Sum/2
  [Tplus] -> Sum1/2
  Gain/1 -> Saturation/1
  Constant1/1 -> Sum/3
  Constant2/1 -> Sum1/3
  Saturation1/1 -> Tminus/1, [Tminus]
  Constant3/1 -> Minus1/1
  Minus1/1 -> Gain1/1
  Integrator/1 -> Minus1/2, Minus/2, Minus2/2, T_mu_mu/1
  Gain1/1 -> Saturation1/1
  [Tminus] -> Sum/4
  [Tminus] -> Sum1/4
  Minus2/1 -> Integrator/1
  Tmean/1 -> Integrator/2, Minus2/1

== system MenakaModel/Control System/PID-set-points/Subsystem1/Heating Controler ==
  In Bus Element : Inport  PortName=EC  Element=Temp
  In Bus Element1 : Inport  Port=2  PortName=IC  Element=Temp.Tair
  u : Inport  Port=3
  Gain : Gain  Gain=power
  Integrator : Integrator  InitialCondition=T  AbsoluteTolerance=0.001
  Sec2Days : Gain  Gain=24*3600
  Subsystem : Subsystem
  Heater : Outport  Unit=J
  Consumptions : Outport  Port=2
  State : Outport  Port=3
  wires:
  Gain/1 -> Consumptions/1, Subsystem/2(Q_h)  "Q_h"
  u/1 -> Gain/1  "Control"
  Sec2Days/1 -> Integrator/1
  In Bus Element1/1 -> Subsystem/1(T_i)
  In Bus Element/1 -> Subsystem/3(T_e)
  Subsystem/1(QV_h_i) -> Heater/1  "QV_h_i"
  Subsystem/2(dT_h_dt) -> Sec2Days/1
  Integrator/1 -> State/1, Subsystem/4(Th)  "Th"

== system MenakaModel/Control System/PID-set-points/Subsystem1/Subsystem2 ==
  Max : Inport
  " Min" : Inport  Port=2
  T : Inport  Port=3
  Gain : Gain
  Gain1 : Gain  Gain=0.05
  Integrator : Integrator
  Minus : Sum  Inputs=+-
  Saturation : Saturate  UpperLimit=1  LowerLimit=0
  Sum : Sum  Inputs=++|
  y : Outport
  wires:
  Max/1 -> ?
  " Min"/1 -> Minus/1
  T/1 -> Minus/2
  Minus/1 -> Integrator/1, Gain/1
  Saturation/1 -> y/1
  Integrator/1 -> Gain1/1
  Gain/1 -> Sum/2
  Sum/1 -> Saturation/1
  Gain1/1 -> Sum/1

== system MenakaModel/Control System/PID-set-points/Subsystem1/Sunset Sunrise ==
  Rad : Inport
  Constant4 : Constant  Value=100
  Gain : Gain  Gain=10
  Minus : Sum  Inputs=+-
  Tan : Trigonometry  Operator=tanh
  Out1 : Outport
  wires:
  Constant4/1 -> Minus/2
  Tan/1 -> Out1/1
  Gain/1 -> Tan/1
  Minus/1 -> Gain/1
  Rad/1 -> Minus/1

== system MenakaModel/Control System/PID-set-points/Subsystem1/Triggered Subsystem ==
  Rad : Inport
  <Tsum> : Inport  Port=2
  Trigger : TriggerPort  TriggerType=either  VariantControl=(inherit)  InitialTriggerSignalState=positive
  Constant : Constant  Value=100
  MATLAB Function : MATLAB Function  TreatAsAtomicUnit=on
  T_min : Outport
  T_opt_min : Outport  Port=2
  T_opt_max : Outport  Port=3
  Tmax : Outport  Port=4
  wires:
  <Tsum>/1 -> MATLAB Function/1(Tsum)
  Rad/1 -> MATLAB Function/2(Rad)
  Constant/1 -> MATLAB Function/3(THRad)
  MATLAB Function/1(T_min) -> T_min/1
  MATLAB Function/2(T_opt_min) -> T_opt_min/1
  MATLAB Function/3(T_opt_max) -> T_opt_max/1
  MATLAB Function/4(Tmax) -> Tmax/1

== system MenakaModel/Control System/PID-set-points/Subsystem1/Windows Controler ==
  note: Subsystem1
  In Bus Element : Inport  PortName=IC  Element=QS.R_int
  In Bus Element1 : Inport  PortName=IC  Element=Temp.Tair
  In Bus Element2 : Inport  PortName=IC  Element=Gas.HRInt
  Tstart : Inport  Port=2
  Tmax : Inport  Port=3
  Hstart : Inport  Port=4
  Hmax : Inport  Port=5
  max_night : Inport  Port=6
  Abs : Abs  ZeroCross=off  SaturateOnIntegerOverflow=off
  Bus Creator : BusCreator  Inputs=2
  Constant : Constant  Value=AR
  Gain : Gain  Gain=100/tau
  Gain1 : Gain  Gain=Power
  Integrator : Integrator
  Minus : Sum  Inputs=+-
  Sec2Days : Gain  Gain=24*3600
  Subsystem : Subsystem
      settings: PortSchema="{\"entries\":[{\"content\":{\"sides\":[{\"content\":{\"connectorIds\":[\"In1\",\"In2\",\"In3\",\"In4\",\"In5\",\"In6\"]},\"type\":\"ConnectorPlacement.EquallySpacedRectSide\",\"uuid\":\"18d05740-181f-409c-94ea-b42b6e57ea74\"},{\"content\":{\"connectorIds\":[\"Out1\"],\"side\":\"RIGHT\"},\"type\":\"ConnectorPlacement.EquallySpacedRectSide\",\"uuid\":\"978406c3-d241-44cd-a3e7-fe734e3a171e\"},{\"content\":{\"connectorIds\":[\"In7\",\"In8\"],\"side\":\"TOP\"},\"type\":\"ConnectorPlacement.EquallySpacedRectSide\",\"uuid\":\"b3c10a0e-c6d9-4444-97f2-9f0c7dea8ec9\"}]},\"type\":\"ConnectorPlacement.EquallySpacedConnector\",\"uuid\":\"429bf3f5-5806-495e-b66b-96810540e6d1\"}],\"packageUris\":[\"http://schema.mathworks.com/mf0/Connector/R2020b\"],\"version\":\"1.0\"}"
  Tanh : Trigonometry  Operator=tanh
  Windows : Outport
  Consumptions : Outport  Port=2
  wires:
  Tstart/1 -> Subsystem/1(Tstart)
  In Bus Element1/1 -> Subsystem/2(Ti)
  Tmax/1 -> Subsystem/3(Tmax)
  Integrator/1 -> Bus Creator/1, Minus/2  "value"
  In Bus Element2/1 -> Subsystem/4(HRInt)
  Hstart/1 -> Subsystem/5(HRStart)
  In Bus Element/1 -> Subsystem/7(Rad)
  Hmax/1 -> Subsystem/6(HRMax)
  Subsystem/1(y) -> Minus/1
  Sec2Days/1 -> Integrator/1
  Gain1/1 -> Consumptions/1  "Power"
  Abs/1 -> Gain1/1
  Gain/1 -> Abs/1, Sec2Days/1
  Tanh/1 -> Gain/1
  Minus/1 -> Tanh/1
  Bus Creator/1 -> Windows/1
  Constant/1 -> Bus Creator/2  "AR"
  max_night/1 -> Subsystem/8(max_night)

== system MenakaModel/Control System/Setpoints Control - ON//OFF/Subsystem/Scalar2Bus  ==
  QV : Inport
  QT : Inport  Port=2
  A : Inport  Port=3
  CC : Inport  Port=4
  Bus Creator : BusCreator  Inputs=4
  CoCl : Outport
  wires:
  A/1 -> Bus Creator/3  "A"
  CC/1 -> Bus Creator/4  "CC"
  QV/1 -> Bus Creator/1  "QV"
  Bus Creator/1 -> CoCl/1
  QT/1 -> Bus Creator/2  "QT"

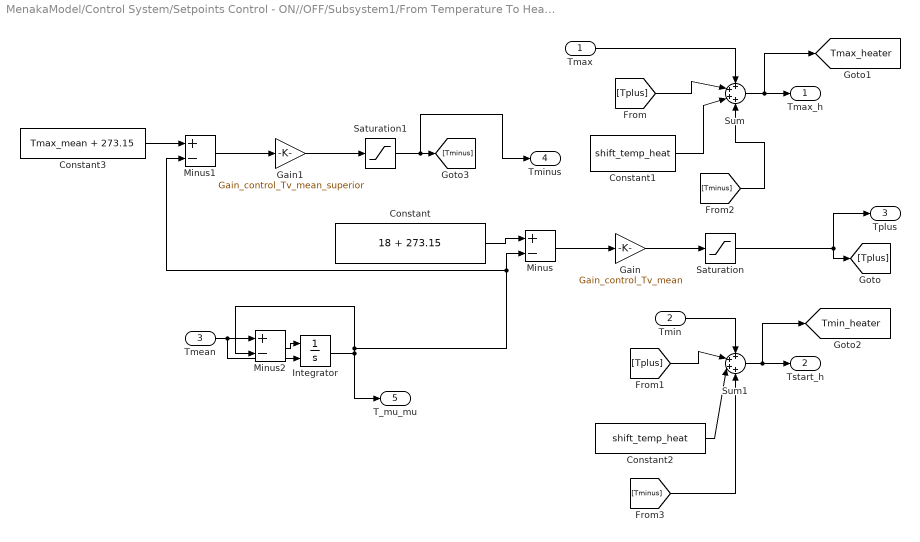
== system MenakaModel/Control System/Setpoints Control - ON//OFF/Subsystem1/From Temperature To Heater ST ==
  Tmax : Inport
  Tmin : Inport  Port=2
  Tmean : Inport  Port=3
  Constant : Constant  Value=18 + 273.15
  Constant1 : Constant  Value=shift_temp_heat
  Constant2 : Constant  Value=shift_temp_heat
  Constant3 : Constant  Value=Tmax_mean + 273.15
  Gain : Gain  Gain=Gain_control_Tv_mean
  Gain1 : Gain  Gain=Gain_control_Tv_mean_superior
  Integrator : Integrator  InitialConditionSource=external
  Minus : Sum  Inputs=+-
  Minus1 : Sum  Inputs=+-
  Minus2 : Sum  Inputs=+-
  Saturation : Saturate  UpperLimit=inf  LowerLimit=0
  Saturation1 : Saturate  UpperLimit=0  LowerLimit=-inf
  Sum : Sum  Inputs=++++
  Sum1 : Sum  Inputs=++++
  Tmax_h : Outport
  Tstart_h : Outport  Port=2
  Tplus : Outport  Port=3
  Tminus : Outport  Port=4
  T_mu_mu : Outport  Port=5
  tag scope: Tmax_heater=global, Tmin_heater=global
  wires:
  Constant/1 -> Minus/1
  Minus/1 -> Gain/1
  Tmax/1 -> Sum/1
  Sum/1 -> [Tmax_heater], Tmax_h/1
  Saturation/1 -> [Tplus], Tplus/1
  Tmin/1 -> Sum1/1
  Sum1/1 -> [Tmin_heater], Tstart_h/1
  [Tplus] -> Sum/2
  [Tplus] -> Sum1/2
  Gain/1 -> Saturation/1
  Constant1/1 -> Sum/3
  Constant2/1 -> Sum1/3
  Saturation1/1 -> Tminus/1, [Tminus]
  Constant3/1 -> Minus1/1
  Minus1/1 -> Gain1/1
  Integrator/1 -> Minus1/2, Minus/2, Minus2/2, T_mu_mu/1
  Gain1/1 -> Saturation1/1
  [Tminus] -> Sum/4
  [Tminus] -> Sum1/4
  Minus2/1 -> Integrator/1
  Tmean/1 -> Integrator/2, Minus2/1

== system MenakaModel/Control System/Setpoints Control - ON//OFF/Subsystem1/Heating Controler ==
  In Bus Element : Inport  PortName=EC  Element=Temp
  In Bus Element1 : Inport  Port=2  PortName=IC  Element=Temp.Tair
  u : Inport  Port=3
  Gain : Gain  Gain=power
  Integrator : Integrator  InitialCondition=T  AbsoluteTolerance=0.001
  Sec2Days : Gain  Gain=24*3600
  Subsystem : Subsystem
  Heater : Outport  Unit=J
  Consumptions : Outport  Port=2
  State : Outport  Port=3
  wires:
  Gain/1 -> Consumptions/1, Subsystem/2(Q_h)  "Q_h"
  u/1 -> Gain/1  "Control"
  Sec2Days/1 -> Integrator/1
  In Bus Element1/1 -> Subsystem/1(T_i)
  In Bus Element/1 -> Subsystem/3(T_e)
  Subsystem/1(QV_h_i) -> Heater/1  "QV_h_i"
  Subsystem/2(dT_h_dt) -> Sec2Days/1
  Integrator/1 -> State/1, Subsystem/4(Th)  "Th"

== system MenakaModel/Control System/Setpoints Control - ON//OFF/Subsystem1/Subsystem2 ==
  Max : Inport
  " Min" : Inport  Port=2
  T : Inport  Port=3
  If : If  NumInputs=3  IfExpression=u2 > u1  ElseIfExpressions=u2 < u3
  If Action Subsystem : Subsystem  TreatAsAtomicUnit=on
  If Action Subsystem1 : Subsystem  TreatAsAtomicUnit=on
  If Action Subsystem2 : Subsystem  TreatAsAtomicUnit=on
  Memory : Memory  InheritSampleTime=on
  Merge : Merge  Inputs=3
  y : Outport
  wires:
  Memory/1 -> If Action Subsystem2/1(In1)
  Merge/1 -> y/1, Memory/1
  If Action Subsystem/1(Out1) -> Merge/1
  If Action Subsystem1/1(Out1) -> Merge/2
  If Action Subsystem2/1(Out1) -> Merge/3
  If/3 -> If Action Subsystem2/Action
  If/2 -> If Action Subsystem1/Action
  If/1 -> If Action Subsystem/Action
  Max/1 -> If/1
  " Min"/1 -> If/3
  T/1 -> If/2

== system MenakaModel/Control System/Setpoints Control - ON//OFF/Subsystem1/Sunset Sunrise ==
  Rad : Inport
  Constant4 : Constant  Value=100
  Gain : Gain  Gain=10
  Minus : Sum  Inputs=+-
  Tan : Trigonometry  Operator=tanh
  Out1 : Outport
  wires:
  Constant4/1 -> Minus/2
  Tan/1 -> Out1/1
  Gain/1 -> Tan/1
  Minus/1 -> Gain/1
  Rad/1 -> Minus/1

== system MenakaModel/Control System/Setpoints Control - ON//OFF/Subsystem1/Triggered Subsystem ==
  Rad : Inport
  <Tsum> : Inport  Port=2
  Trigger : TriggerPort  TriggerType=either  VariantControl=(inherit)  InitialTriggerSignalState=positive
  Constant : Constant  Value=100
  MATLAB Function : MATLAB Function  TreatAsAtomicUnit=on
  T_min : Outport
  T_opt_min : Outport  Port=2
  T_opt_max : Outport  Port=3
  Tmax : Outport  Port=4
  wires:
  <Tsum>/1 -> MATLAB Function/1(Tsum)
  Rad/1 -> MATLAB Function/2(Rad)
  Constant/1 -> MATLAB Function/3(THRad)
  MATLAB Function/1(T_min) -> T_min/1
  MATLAB Function/2(T_opt_min) -> T_opt_min/1
  MATLAB Function/3(T_opt_max) -> T_opt_max/1
  MATLAB Function/4(Tmax) -> Tmax/1

== system MenakaModel/Control System/Setpoints Control - ON//OFF/Subsystem1/Windows Controler ==
  note: Subsystem1
  In Bus Element : Inport  PortName=IC  Element=QS.R_int
  In Bus Element1 : Inport  PortName=IC  Element=Temp.Tair
  In Bus Element2 : Inport  PortName=IC  Element=Gas.HRInt
  Tstart : Inport  Port=2
  Tmax : Inport  Port=3
  Hstart : Inport  Port=4
  Hmax : Inport  Port=5
  max_night : Inport  Port=6
  Abs : Abs  ZeroCross=off  SaturateOnIntegerOverflow=off
  Bus Creator : BusCreator  Inputs=2
  Constant : Constant  Value=AR
  Gain : Gain  Gain=100/tau
  Gain1 : Gain  Gain=Power
  Integrator : Integrator
  Minus : Sum  Inputs=+-
  Sec2Days : Gain  Gain=24*3600
  Subsystem : Subsystem
      settings: PortSchema="{\"entries\":[{\"content\":{\"sides\":[{\"content\":{\"connectorIds\":[\"In1\",\"In2\",\"In3\",\"In4\",\"In5\",\"In6\"]},\"type\":\"ConnectorPlacement.EquallySpacedRectSide\",\"uuid\":\"18d05740-181f-409c-94ea-b42b6e57ea74\"},{\"content\":{\"connectorIds\":[\"Out1\"],\"side\":\"RIGHT\"},\"type\":\"ConnectorPlacement.EquallySpacedRectSide\",\"uuid\":\"978406c3-d241-44cd-a3e7-fe734e3a171e\"},{\"content\":{\"connectorIds\":[\"In7\",\"In8\"],\"side\":\"TOP\"},\"type\":\"ConnectorPlacement.EquallySpacedRectSide\",\"uuid\":\"b3c10a0e-c6d9-4444-97f2-9f0c7dea8ec9\"}]},\"type\":\"ConnectorPlacement.EquallySpacedConnector\",\"uuid\":\"429bf3f5-5806-495e-b66b-96810540e6d1\"}],\"packageUris\":[\"http://schema.mathworks.com/mf0/Connector/R2020b\"],\"version\":\"1.0\"}"
  Tanh : Trigonometry  Operator=tanh
  Windows : Outport
  Consumptions : Outport  Port=2
  wires:
  Tstart/1 -> Subsystem/1(Tstart)
  In Bus Element1/1 -> Subsystem/2(Ti)
  Tmax/1 -> Subsystem/3(Tmax)
  Integrator/1 -> Bus Creator/1, Minus/2  "value"
  In Bus Element2/1 -> Subsystem/4(HRInt)
  Hstart/1 -> Subsystem/5(HRStart)
  In Bus Element/1 -> Subsystem/7(Rad)
  Hmax/1 -> Subsystem/6(HRMax)
  Subsystem/1(y) -> Minus/1
  Sec2Days/1 -> Integrator/1
  Gain1/1 -> Consumptions/1  "Power"
  Abs/1 -> Gain1/1
  Gain/1 -> Abs/1, Sec2Days/1
  Tanh/1 -> Gain/1
  Minus/1 -> Tanh/1
  Bus Creator/1 -> Windows/1
  Constant/1 -> Bus Creator/2  "AR"
  max_night/1 -> Subsystem/8(max_night)

== system MenakaModel/Subsystem1/For Each Subsystem/Subsystem/If Action Subsystem ==
  Action Port : ActionPort  ActionPortLabel=if(u1 < 1e-9)
  Constant : Constant  Value=0
  Constant1 : Constant  Value=0
  Out1 : Outport
  Out2 : Outport  Port=2
  wires:
  Constant/1 -> Out1/1
  Constant1/1 -> Out2/1

== system MenakaModel/Subsystem1/For Each Subsystem/Subsystem/If Action Subsystem1 ==
  In1 : Inport
  In2 : Inport  Port=2
  In3 : Inport  Port=3
  Action Port : ActionPort  ActionPortLabel=else
  Divide : Product  Inputs=*/
  Divide1 : Product  Inputs=*/
  Out1 : Outport
  Out2 : Outport  Port=2
  wires:
  In1/1 -> Divide/1
  In2/1 -> Divide1/1
  In3/1 -> Divide1/2, Divide/2
  Divide/1 -> Out1/1
  Divide1/1 -> Out2/1

== system MenakaModel/Control System/Control System Proportional (Ti) + Tmu /Heating Controler/Subsystem/Subsystem1 ==
  Ti : Inport
  A_h_exp : Inport  Port=2
  Th : Inport  Port=3
  Divide2 : Product  Inputs=****/
  Subsystem : Subsystem
  d_h1 : Constant  Value=1.5
  lambda thermal conductivity of air [W/m/K] : Constant  Value=0.025
  QV_h_i : Outport
  wires:
  Divide2/1 -> QV_h_i/1
  Subsystem/2(dT) -> Divide2/4
  Subsystem/1(Gr) -> Divide2/2
  d_h1/1 -> Divide2/5
  A_h_exp/1 -> Divide2/3
  lambda thermal conductivity of air [W/m/K]/1 -> Divide2/1
  Th/1 -> Subsystem/2(Th)
  Ti/1 -> Subsystem/1(Ti)

== system MenakaModel/Control System/Control System Proportional (Ti) + Tmu /Heating Controler/Subsystem/Subsystem2 ==
  Te : Inport
  A_h_exp : Inport  Port=2
  Th : Inport  Port=3
  Divide2 : Product  Inputs=****/
  Subsystem : Subsystem
  d_h1 : Constant  Value=1.5
  lambda thermal conductivity of air [W/m/K] : Constant  Value=0.025
  QV_h_e : Outport
  wires:
  Divide2/1 -> QV_h_e/1
  Subsystem/2(dT) -> Divide2/4
  Subsystem/1(Gr) -> Divide2/2
  d_h1/1 -> Divide2/5
  A_h_exp/1 -> Divide2/3
  lambda thermal conductivity of air [W/m/K]/1 -> Divide2/1
  Th/1 -> Subsystem/2(Th)
  Te/1 -> Subsystem/1(Ti)

== system MenakaModel/Control System/Control System Proportional (Ti) + Tmu /Selector/Windows Controler/Subsystem ==
  Tstart : Inport
  Ti : Inport  Port=2
  Tmax : Inport  Port=3
  HRInt : Inport  Port=4
  HRStart : Inport  Port=5
  HRMax : Inport  Port=6
  Rad : Inport  Port=7
  Constant : Constant  Value=RadThreshold
  Hum : Saturate  UpperLimit=max_night  LowerLimit=0
  "Selection " : MATLAB Function  TreatAsAtomicUnit=on
  Temp : Saturate  UpperLimit=100  LowerLimit=0
  Ventilation by Hight Humidity : MATLAB Function  TreatAsAtomicUnit=on
  Ventilation by Hight Temperature1 : MATLAB Function  TreatAsAtomicUnit=on
  y : Outport
  wires:
  Ti/1 -> Ventilation by Hight Temperature1/2(Ti)
  Rad/1 -> "Selection "/1(Rad)
  Tstart/1 -> Ventilation by Hight Temperature1/1(Tstart)
  Hum/1 -> "Selection "/3(Humidity)
  HRMax/1 -> Ventilation by Hight Humidity/3(HRMax)
  Tmax/1 -> Ventilation by Hight Temperature1/3(Tmax)
  "Selection "/1(y) -> y/1
  Ventilation by Hight Humidity/1(y) -> Hum/1
  HRStart/1 -> Ventilation by Hight Humidity/2(HRStart)
  Ventilation by Hight Temperature1/1(y) -> Temp/1
  HRInt/1 -> Ventilation by Hight Humidity/1(HRInt)
  Temp/1 -> "Selection "/2(Temperature)
  Constant/1 -> "Selection "/4(Rad_threshold)

== system MenakaModel/Control System/Control System Proportional (Ti) + Tmu Windows Relay/Heating Controler/Subsystem/Subsystem1 ==
  Ti : Inport
  A_h_exp : Inport  Port=2
  Th : Inport  Port=3
  Divide2 : Product  Inputs=****/
  Subsystem : Subsystem
  d_h1 : Constant  Value=1.5
  lambda thermal conductivity of air [W/m/K] : Constant  Value=0.025
  QV_h_i : Outport
  wires:
  Divide2/1 -> QV_h_i/1
  Subsystem/2(dT) -> Divide2/4
  Subsystem/1(Gr) -> Divide2/2
  d_h1/1 -> Divide2/5
  A_h_exp/1 -> Divide2/3
  lambda thermal conductivity of air [W/m/K]/1 -> Divide2/1
  Th/1 -> Subsystem/2(Th)
  Ti/1 -> Subsystem/1(Ti)

== system MenakaModel/Control System/Control System Proportional (Ti) + Tmu Windows Relay/Heating Controler/Subsystem/Subsystem2 ==
  Te : Inport
  A_h_exp : Inport  Port=2
  Th : Inport  Port=3
  Divide2 : Product  Inputs=****/
  Subsystem : Subsystem
  d_h1 : Constant  Value=1.5
  lambda thermal conductivity of air [W/m/K] : Constant  Value=0.025
  QV_h_e : Outport
  wires:
  Divide2/1 -> QV_h_e/1
  Subsystem/2(dT) -> Divide2/4
  Subsystem/1(Gr) -> Divide2/2
  d_h1/1 -> Divide2/5
  A_h_exp/1 -> Divide2/3
  lambda thermal conductivity of air [W/m/K]/1 -> Divide2/1
  Th/1 -> Subsystem/2(Th)
  Te/1 -> Subsystem/1(Ti)

== system MenakaModel/Control System/Control System Proportional (Ti) + Tmu Windows Relay/Screen Controler/Subsystem/If Action Subsystem ==
  Action Port : ActionPort  ActionPortLabel=if(u1 < 10)
  Constant : Constant  Value=100
  Out1 : Outport
  wires:
  Constant/1 -> Out1/1

== system MenakaModel/Control System/Control System Proportional (Ti) + Tmu Windows Relay/Screen Controler/Subsystem/If Action Subsystem1 ==
  EC : Inport
  Radthhold : Inport  Port=2
  Action Port : ActionPort  ActionPortLabel=else
  Gain1 : Gain  Gain=100
  Minus1 : Sum  Inputs=+-
  "Theta " : Subsystem
  Out1 : Outport
  wires:
  "Theta "/1(Out1) -> Gain1/1
  Minus1/1 -> "Theta "/1(In1)
  EC/1 -> Minus1/1
  Gain1/1 -> Out1/1
  Radthhold/1 -> Minus1/2

== system MenakaModel/Control System/Control System Proportional (Ti) + Tmu Windows Relay/Screen Controler/Subsystem/Smooth Rad ==
  In1 : Inport
  Integrator1 : Integrator
  Minus2 : Sum  Inputs=+-
  Sec2Days1 : Gain  Gain=24*3600
  Out1 : Outport
  wires:
  In1/1 -> Minus2/1
  Sec2Days1/1 -> Integrator1/1
  Minus2/1 -> Sec2Days1/1
  Integrator1/1 -> Out1/1, Minus2/2
